simulink library "QRS_Detector_Library"  (R2021a)
settings: Solver=VariableStepAuto  StartTime=0.0  StopTime=10.0  RelTol=1e-3
undefined symbols (not defined in the file): centerFrequency, qualityFactor, sampleTime
libraries: simulink x2
settings Model: Creator=wallyproenza  LastModifiedBy=wallyproenza

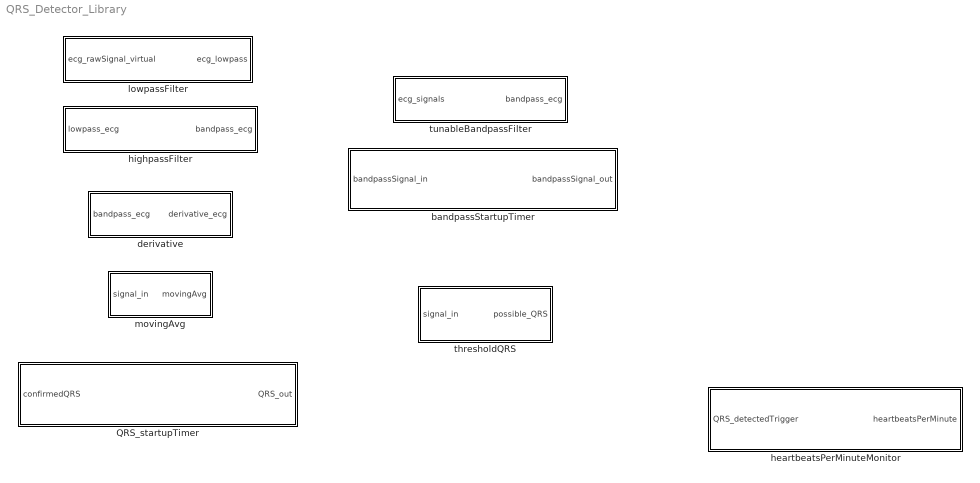
== system QRS_Detector_Library ==
  QRS_startupTimer : Subsystem
  bandpassStartupTimer : Subsystem
  derivative : Subsystem
  heartbeatsPerMinuteMonitor : Subsystem
  highpassFilter : Subsystem
  lowpassFilter : Subsystem
  movingAvg : Subsystem
  thresholdQRS : Subsystem
  tunableBandpassFilter : Subsystem

== system QRS_Detector_Library/QRS_startupTimer ==
  note: QRS startup timer helps avoid startup-related false positives
  confirmedQRS : Inport
  Cast To Double1 : DataTypeConversion  OutDataTypeStr=double
  Clock1 : Clock
  Switch1 : Switch  Criteria=u2 > Threshold  Threshold=900*sampleTime
  Zero1 : Constant  Value=0  OutDataTypeStr=Inherit: Inherit via back propagation
  QRS_out : Outport
  wires:
  confirmedQRS/1 -> Switch1/1
  Zero1/1 -> Switch1/3
  Cast To Double1/1 -> Switch1/2
  Switch1/1 -> QRS_out/1
  Clock1/1 -> Cast To Double1/1

== system QRS_Detector_Library/bandpassStartupTimer ==
  note: This bandpass startup timer helps avoids startup-related noise skew
  bandpassSignal_in : Inport
  Cast To Double : DataTypeConversion  OutDataTypeStr=double
  Clock : Clock
  Switch : Switch  Criteria=u2 > Threshold  Threshold=125*sampleTime
  Zero : Constant  Value=0  OutDataTypeStr=Inherit: Inherit via back propagation
  bandpassSignal_out : Outport
  wires:
  Cast To Double/1 -> Switch/2
  Switch/1 -> bandpassSignal_out/1
  bandpassSignal_in/1 -> Switch/1
  Zero/1 -> Switch/3
  Clock/1 -> Cast To Double/1

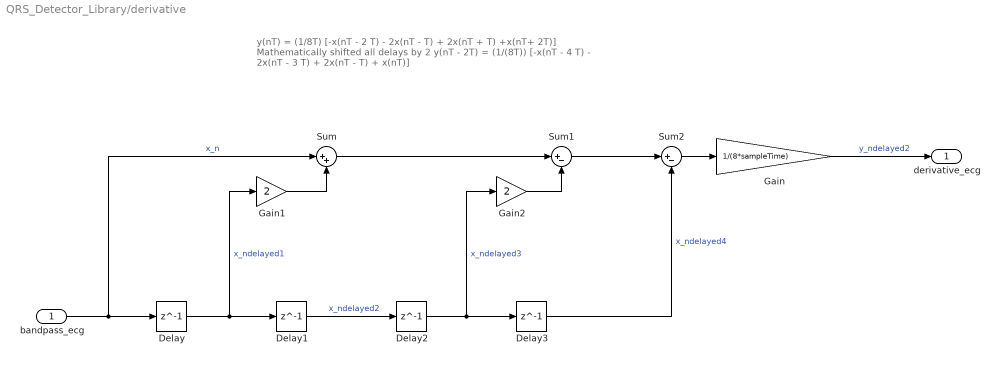
== system QRS_Detector_Library/derivative ==
  note: y(nT) = (1/8T) [-x(nT - 2 T) - 2x(nT - T) + 2x(nT + T) +x(nT+ 2T)]
      |
      | Mathematically shifted all delays by 2
      |
      | y(nT - 2T) = (1/(8T)) [-x(nT - 4 T) - 2x(nT - 3 T) + 2x(nT - T) + x(nT)]
  bandpass_ecg : Inport
  Delay{,1..3} (4 alike) : Delay  DelayLength=1  InitialCondition=0
  Gain : Gain  Gain=1/(8*sampleTime)
  Gain1 : Gain  Gain=2
  Gain2 : Gain  Gain=2
  Sum : Sum  Inputs=|++
  Sum1 : Sum  Inputs=|+-
  Sum2 : Sum  Inputs=|+-
  derivative_ecg : Outport
  wires:
  Gain/1 -> derivative_ecg/1  "y_ndelayed2"
  bandpass_ecg/1 -> Sum/1, Delay/1  "x_n"
  Delay/1 -> Gain1/1, Delay1/1  "x_ndelayed1"
  Delay1/1 -> Delay2/1  "x_ndelayed2"
  Delay2/1 -> Gain2/1, Delay3/1  "x_ndelayed3"
  Delay3/1 -> Sum2/2  "x_ndelayed4"
  Gain1/1 -> Sum/2
  Gain2/1 -> Sum1/2
  Sum/1 -> Sum1/1
  Sum1/1 -> Sum2/1
  Sum2/1 -> Gain/1

== system QRS_Detector_Library/heartbeatsPerMinuteMonitor ==
  QRS_detectedTrigger : Inport
  Cast To Double : DataTypeConversion  OutDataTypeStr=double
  Clock1 : Clock
  Compare To Constant : simulink/Logic and Bit Operations/Compare To Constant  relop=>=  const=900*sampleTime  OutDataTypeStr=boolean
  Enabled and Triggered Subsystem : Subsystem  TreatAsAtomicUnit=on
  heartbeatsPerMinute : Outport
  wires:
  QRS_detectedTrigger/1 -> Enabled and Triggered Subsystem/Trigger, Enabled and Triggered Subsystem/2(QRS_detectedTrigger)
  Clock1/1 -> Cast To Double/1
  Enabled and Triggered Subsystem/1(heartbeatsPerMinute) -> heartbeatsPerMinute/1
  Compare To Constant/1 -> Enabled and Triggered Subsystem/Enable
  Cast To Double/1 -> Enabled and Triggered Subsystem/1(clock), Compare To Constant/1

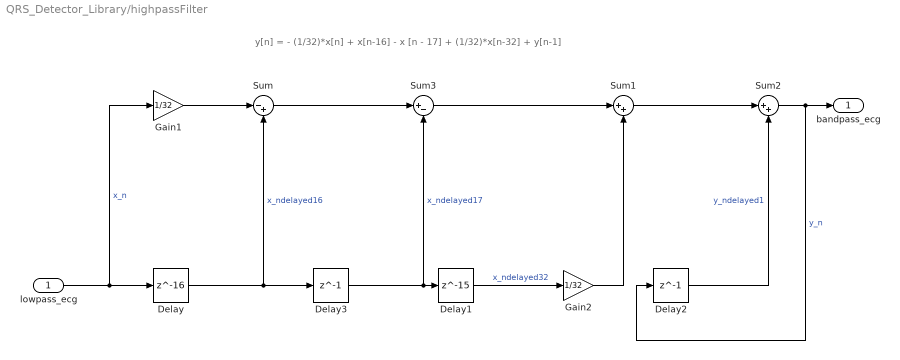
== system QRS_Detector_Library/highpassFilter ==
  note: y[n] = - (1/32)*x[n] + x[n-16] - x [n - 17] + (1/32)*x[n-32] + y[n-1]
  lowpass_ecg : Inport
  Delay : Delay  DelayLength=16  InitialCondition=0
  Delay1 : Delay  DelayLength=15  InitialCondition=0
  Delay2 : Delay  DelayLength=1  InitialCondition=0
  Delay3 : Delay  DelayLength=1  InitialCondition=0
  Gain1 : Gain  Gain=1/32
  Gain2 : Gain  Gain=1/32
  Sum : Sum  Inputs=|-+
  Sum1 : Sum  Inputs=|++
  Sum2 : Sum  Inputs=|++
  Sum3 : Sum  Inputs=|+-
  bandpass_ecg : Outport
  wires:
  lowpass_ecg/1 -> Gain1/1, Delay/1  "x_n"
  Delay/1 -> Delay3/1, Sum/2  "x_ndelayed16"
  Delay1/1 -> Gain2/1  "x_ndelayed32"
  Sum1/1 -> Sum2/1
  Delay2/1 -> Sum2/2  "y_ndelayed1"
  Sum2/1 -> Delay2/1, bandpass_ecg/1  "y_n"
  Gain1/1 -> Sum/1
  Delay3/1 -> Delay1/1, Sum3/2  "x_ndelayed17"
  Sum/1 -> Sum3/1
  Sum3/1 -> Sum1/1
  Gain2/1 -> Sum1/2

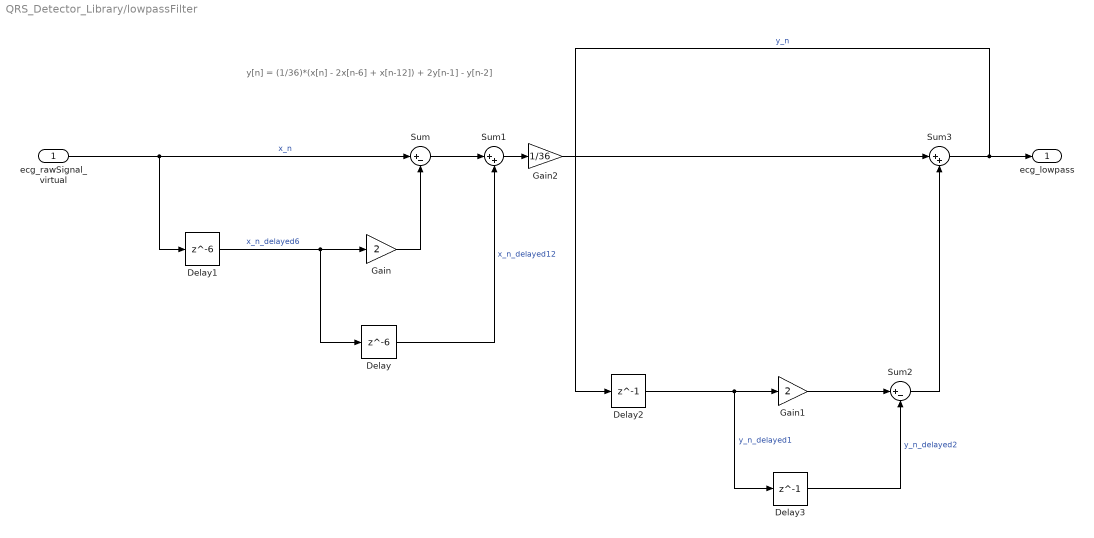
== system QRS_Detector_Library/lowpassFilter ==
  note: y[n] = (1/36)*(x[n] - 2x[n-6] + x[n-12]) + 2y[n-1] - y[n-2]
  ecg_rawSignal_virtual : Inport
  Delay : Delay  DelayLength=6  InitialCondition=0
  Delay1 : Delay  DelayLength=6  InitialCondition=0
  Delay2 : Delay  DelayLength=1  InitialCondition=0
  Delay3 : Delay  DelayLength=1  InitialCondition=0
  Gain : Gain  Gain=2
  Gain1 : Gain  Gain=2
  Gain2 : Gain  Gain=1/36
  Sum : Sum  Inputs=|+-
  Sum1 : Sum  Inputs=|++
  Sum2 : Sum  Inputs=|+-
  Sum3 : Sum  Inputs=|++
  ecg_lowpass : Outport
  wires:
  ecg_rawSignal_virtual/1 -> Delay1/1, Sum/1  "x_n"
  Delay1/1 -> Gain/1, Delay/1  "x_n_delayed6"
  Gain/1 -> Sum/2
  Delay/1 -> Sum1/2  "x_n_delayed12"
  Sum/1 -> Sum1/1
  Sum1/1 -> Gain2/1
  Delay2/1 -> Delay3/1, Gain1/1  "y_n_delayed1"
  Gain1/1 -> Sum2/1
  Delay3/1 -> Sum2/2  "y_n_delayed2"
  Sum2/1 -> Sum3/2
  Sum3/1 -> ecg_lowpass/1, Delay2/1  "y_n"
  Gain2/1 -> Sum3/1

== system QRS_Detector_Library/movingAvg ==
  signal_in : Inport
  Add : Sum  Inputs=+-+
  Constant : Constant  Value=38
  Delay : Delay  DelayLength=38  InitialCondition=0
  Delay1 : Delay  DelayLength=1  InitialCondition=0
  Divide : Product  Inputs=*/
  movingAvg : Outport
  wires:
  Constant/1 -> Divide/2
  Divide/1 -> movingAvg/1
  signal_in/1 -> Delay/1, Add/1  "x_n"
  Delay/1 -> Add/2  "x_ndelayed38"
  Add/1 -> Divide/1, Delay1/1  "currSum"
  Delay1/1 -> Add/3  "prevSum"

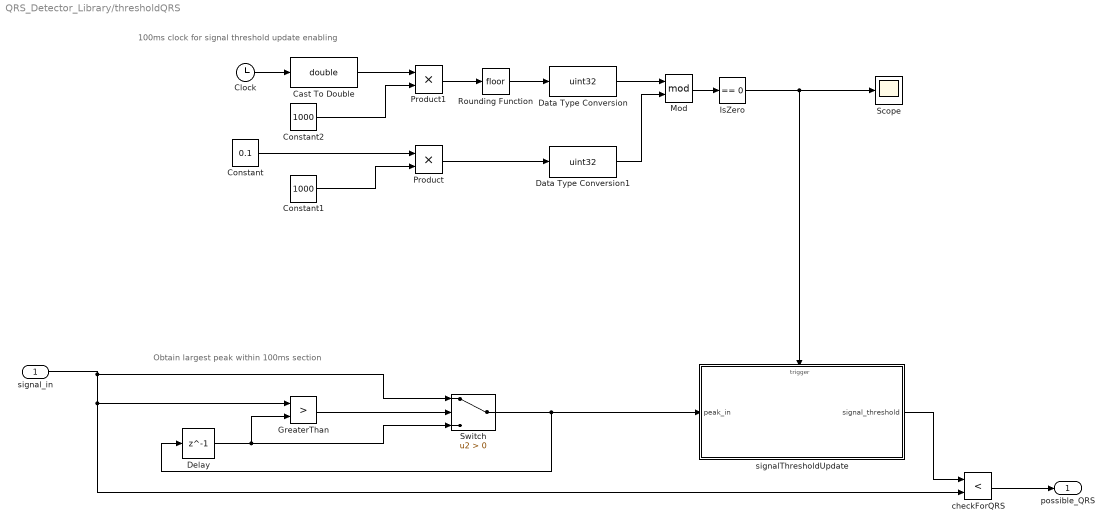
== system QRS_Detector_Library/thresholdQRS ==
  note: Obtain largest peak within 100ms section
  note: 100ms clock for signal threshold update enabling
  signal_in : Inport
  Cast To Double : DataTypeConversion  OutDataTypeStr=double
  Clock : Clock
  Constant : Constant  Value=0.1
  Constant1 : Constant  Value=1000
  Constant2 : Constant  Value=1000
  Data Type Conversion : DataTypeConversion  OutDataTypeStr=uint32
  Data Type Conversion1 : DataTypeConversion  OutDataTypeStr=uint32
  Delay : Delay  DelayLength=1  InitialCondition=0
  GreaterThan : RelationalOperator  Operator=>  OutDataTypeStr=boolean  RndMeth=Simplest
  IsZero : simulink/Logic and Bit Operations/Compare To Zero  relop===  OutDataTypeStr=boolean
  Mod : Math  Operator=mod  SaturateOnIntegerOverflow=on
  Product : Product
  Product1 : Product
  Rounding Function : Rounding
  Scope : Scope
  Switch : Switch  Criteria=u2 > Threshold
  checkForQRS : RelationalOperator  Operator=<  OutDataTypeStr=boolean  RndMeth=Simplest
  signalThresholdUpdate : Subsystem
  possible_QRS : Outport
  wires:
  signal_in/1 -> checkForQRS/2, GreaterThan/1, Switch/1
  signalThresholdUpdate/1(signal_threshold) -> checkForQRS/1
  Rounding Function/1 -> Data Type Conversion/1
  Constant/1 -> Product/1
  Product/1 -> Data Type Conversion1/1
  Constant1/1 -> Product/2
  Constant2/1 -> Product1/2
  Clock/1 -> Cast To Double/1
  Product1/1 -> Rounding Function/1
  Data Type Conversion1/1 -> Mod/2
  Data Type Conversion/1 -> Mod/1
  Mod/1 -> IsZero/1
  IsZero/1 -> signalThresholdUpdate/Trigger, Scope/1
  Cast To Double/1 -> Product1/1
  checkForQRS/1 -> possible_QRS/1
  GreaterThan/1 -> Switch/2
  Switch/1 -> Delay/1, signalThresholdUpdate/1(peak_in)
  Delay/1 -> Switch/3, GreaterThan/2

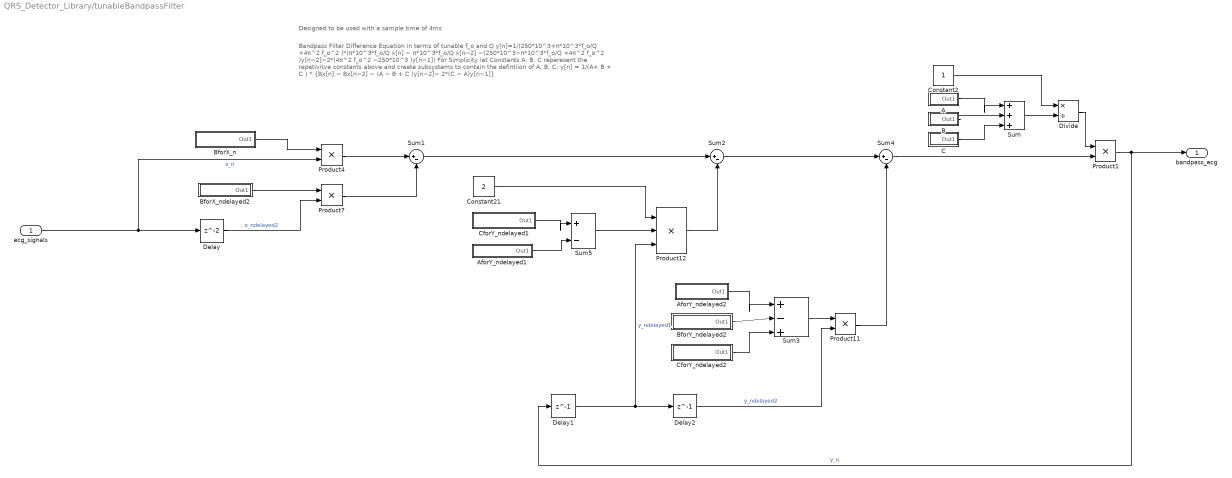
== system QRS_Detector_Library/tunableBandpassFilter ==
  note: Bandpass Filter Difference Equation in terms of tunable f_o and Q
      |
      | y[n]=1/(250*10^3+π*10^3*f_o/Q  +4π^2 f_o^2 )*(π*10^3*f_o/Q x[n]  − π*10^3*f_o/Q x[n−2]  −(250*10^3−π*10^3*f_o/Q  +4π^2 f_o^2 )y[n−2]−2*(4π^2 f_o^2  −250*10^3 )y[n−1])
      |
      |
      | For Simplicity let Constants A, B, C reperesent the repetivitve constants above and create subsystems to contain the defintiion of A, B, C:
      |
      | y[n] = 1/(A+ B + C ) * {Bx[n]  − Bx[n−2]  − (A − B + C )y[n−2]− 2*(C  − A)y[n−1]}
  note: Designed to be used with a sample time of 4ms
  ecg_signals : Inport
  A : Subsystem
  AforY_ndelayed1 : Subsystem
  AforY_ndelayed2 : Subsystem
  B : Subsystem
  BforX_n : Subsystem
  BforX_ndelayed2 : Subsystem
  BforY_ndelayed2 : Subsystem
  C : Subsystem
  CforY_ndelayed1 : Subsystem
  CforY_ndelayed2 : Subsystem
  Constant2 : Constant
  Constant21 : Constant  Value=2
  Delay : Delay  InitialCondition=0
  Delay1 : Delay  DelayLength=1  InitialCondition=0
  Delay2 : Delay  DelayLength=1  InitialCondition=0
  Divide : Product  Inputs=*/
  Product{1,4,7,11} (4 alike) : Product
  Product12 : Product  Inputs=3
  Sum : Sum  Inputs=|+++
  Sum{1..2,4..5} (4 alike) : Sum  Inputs=|+-
  Sum3 : Sum  Inputs=|+-+
  bandpass_ecg : Outport
  wires:
  ecg_signals/1 -> Product4/2, Delay/1  "x_n"
  Delay1/1 -> Product12/3, Delay2/1  "y_ndelayed1"
  Product1/1 -> Delay1/1, bandpass_ecg/1  "y_n"
  Constant2/1 -> Divide/1
  Sum/1 -> Divide/2
  Divide/1 -> Product1/1
  Product4/1 -> Sum1/1
  Product7/1 -> Sum1/2
  Delay/1 -> Product7/2  "x_ndelayed2"
  Sum1/1 -> Sum2/1
  Sum3/1 -> Product11/1
  Product11/1 -> Sum4/2
  Delay2/1 -> Product11/2  "y_ndelayed2"
  Sum4/1 -> Product1/2
  Sum2/1 -> Sum4/1
  Product12/1 -> Sum2/2
  Constant21/1 -> Product12/1
  Sum5/1 -> Product12/2
  A/1(Out1) -> Sum/1
  B/1(Out1) -> Sum/2
  C/1(Out1) -> Sum/3
  BforX_n/1(Out1) -> Product4/1
  BforX_ndelayed2/1(Out1) -> Product7/1
  AforY_ndelayed1/1(Out1) -> Sum5/2
  CforY_ndelayed1/1(Out1) -> Sum5/1
  AforY_ndelayed2/1(Out1) -> Sum3/1
  BforY_ndelayed2/1(Out1) -> Sum3/2
  CforY_ndelayed2/1(Out1) -> Sum3/3

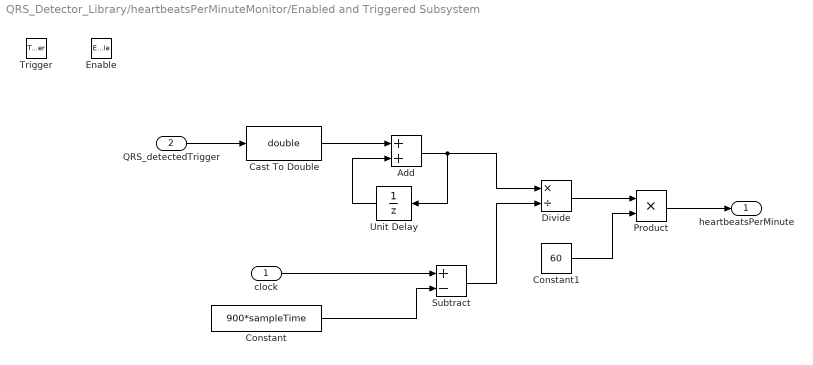
== system QRS_Detector_Library/heartbeatsPerMinuteMonitor/Enabled and Triggered Subsystem ==
  clock : Inport
  QRS_detectedTrigger : Inport  Port=2
  Enable : EnablePort
  Trigger : TriggerPort  VariantControl=(inherit)
  Add : Sum
  Cast To Double : DataTypeConversion  OutDataTypeStr=double
  Constant : Constant  Value=900*sampleTime
  Constant1 : Constant  Value=60
  Divide : Product  Inputs=*/
  Product : Product
  Subtract : Sum  Inputs=+-
  Unit Delay : UnitDelay  SampleTime=-1  HasFrameUpgradeWarning=on
  heartbeatsPerMinute : Outport
  wires:
  clock/1 -> Subtract/1
  Constant/1 -> Subtract/2
  Constant1/1 -> Product/2
  Subtract/1 -> Divide/2
  Product/1 -> heartbeatsPerMinute/1
  QRS_detectedTrigger/1 -> Cast To Double/1
  Add/1 -> Unit Delay/1, Divide/1
  Unit Delay/1 -> Add/2
  Divide/1 -> Product/1
  Cast To Double/1 -> Add/1

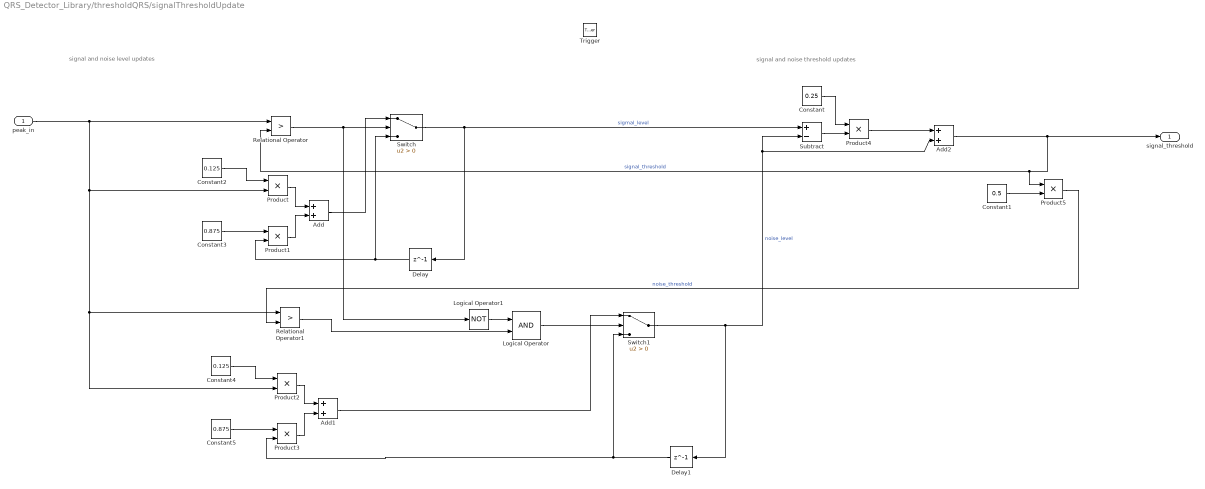
== system QRS_Detector_Library/thresholdQRS/signalThresholdUpdate ==
  note: signal and noise threshold updates
  note: signal and noise level updates
  peak_in : Inport
  Trigger : TriggerPort  VariantControl=(inherit)  PortDimensions=1
  Add : Sum
  Add1 : Sum
  Add2 : Sum
  Constant : Constant  Value=0.25
  Constant1 : Constant  Value=0.5
  Constant2 : Constant  Value=0.125
  Constant3 : Constant  Value=0.875
  Constant4 : Constant  Value=0.125
  Constant5 : Constant  Value=0.875
  Delay : Delay  DelayLength=1  InitialCondition=0
  Delay1 : Delay  DelayLength=1  InitialCondition=0
  Logical Operator : Logic  IconShape=distinctive  AllPortsSameDT=off  OutDataTypeStr=boolean
  Logical Operator1 : Logic  Operator=NOT  IconShape=distinctive  AllPortsSameDT=off  OutDataTypeStr=boolean
  Product{,1..5} (6 alike) : Product
  Relational Operator : RelationalOperator  Operator=>  OutDataTypeStr=boolean  RndMeth=Simplest
  Relational Operator1 : RelationalOperator  Operator=>  OutDataTypeStr=boolean  RndMeth=Simplest
  Subtract : Sum  Inputs=+-
  Switch : Switch  Criteria=u2 > Threshold
  Switch1 : Switch  Criteria=u2 > Threshold
  signal_threshold : Outport
  wires:
  Constant5/1 -> Product3/1
  Product3/1 -> Add1/2
  Add/1 -> Switch/1
  Product2/1 -> Add1/1
  Switch1/1 -> Delay1/1, Add2/2, Subtract/2  "noise_level"
  Product/1 -> Add/1
  Constant2/1 -> Product/1
  Constant1/1 -> Product5/2
  Add2/1 -> signal_threshold/1, Product5/1, Relational Operator/2  "signal_threshold"
  Product4/1 -> Add2/1
  Logical Operator/1 -> Switch1/2
  Constant/1 -> Product4/1
  peak_in/1 -> Relational Operator/1, Product/2, Relational Operator1/1, Product2/2
  Delay1/1 -> Product3/2, Switch1/3
  Logical Operator1/1 -> Logical Operator/1
  Constant4/1 -> Product2/1
  Delay/1 -> Switch/3, Product1/2
  Product1/1 -> Add/2
  Add1/1 -> Switch1/1
  Switch/1 -> Delay/1, Subtract/1  "sigmal_level"
  Constant3/1 -> Product1/1
  Relational Operator/1 -> Logical Operator1/1, Switch/2
  Product5/1 -> Relational Operator1/2  "noise_threshold"
  Subtract/1 -> Product4/2
  Relational Operator1/1 -> Logical Operator/2

== system QRS_Detector_Library/tunableBandpassFilter/A ==
  Constant : Constant  Value=250
  Constant1 : Constant  Value=3
  Power of 10 : Math  Operator=10^u  SaturateOnIntegerOverflow=on
  Product : Product
  Out1 : Outport
  wires:
  Power of 10/1 -> Product/2
  Constant/1 -> Product/1
  Product/1 -> Out1/1
  Constant1/1 -> Power of 10/1

== system QRS_Detector_Library/tunableBandpassFilter/AforY_ndelayed1 ==
  Constant24 : Constant  Value=250
  Constant25 : Constant  Value=3
  Power of 6 : Math  Operator=10^u  SaturateOnIntegerOverflow=on
  Product14 : Product
  Out1 : Outport
  wires:
  Product14/1 -> Out1/1
  Power of 6/1 -> Product14/2
  Constant24/1 -> Product14/1
  Constant25/1 -> Power of 6/1

== system QRS_Detector_Library/tunableBandpassFilter/AforY_ndelayed2 ==
  Constant14 : Constant  Value=250
  Constant15 : Constant  Value=3
  Power of 5 : Math  Operator=10^u  SaturateOnIntegerOverflow=on
  Product8 : Product
  Out1 : Outport
  wires:
  Constant14/1 -> Product8/1
  Product8/1 -> Out1/1
  Power of 5/1 -> Product8/2
  Constant15/1 -> Power of 5/1

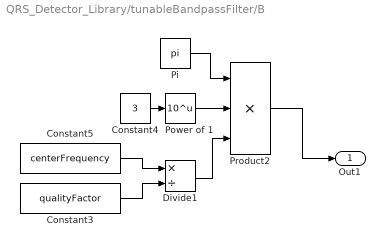
== system QRS_Detector_Library/tunableBandpassFilter/B ==
  Constant3 : Constant  Value=qualityFactor
  Constant4 : Constant  Value=3
  Constant5 : Constant  Value=centerFrequency
  Divide1 : Product  Inputs=*/
  Pi : Constant  Value=pi  OutDataTypeStr=Inherit: Inherit via back propagation
  Power of 1 : Math  Operator=10^u  SaturateOnIntegerOverflow=on
  Product2 : Product  Inputs=3
  Out1 : Outport
  wires:
  Product2/1 -> Out1/1
  Constant5/1 -> Divide1/1
  Divide1/1 -> Product2/3
  Power of 1/1 -> Product2/2
  Constant3/1 -> Divide1/2
  Pi/1 -> Product2/1
  Constant4/1 -> Power of 1/1

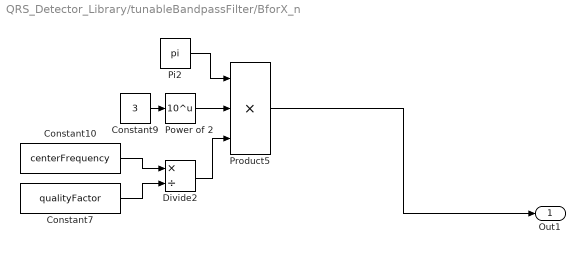
== system QRS_Detector_Library/tunableBandpassFilter/BforX_n ==
  Constant10 : Constant  Value=centerFrequency
  Constant7 : Constant  Value=qualityFactor
  Constant9 : Constant  Value=3
  Divide2 : Product  Inputs=*/
  Pi2 : Constant  Value=pi  OutDataTypeStr=Inherit: Inherit via back propagation
  Power of 2 : Math  Operator=10^u  SaturateOnIntegerOverflow=on
  Product5 : Product  Inputs=3
  Out1 : Outport
  wires:
  Product5/1 -> Out1/1
  Divide2/1 -> Product5/3
  Constant7/1 -> Divide2/2
  Constant10/1 -> Divide2/1
  Pi2/1 -> Product5/1
  Constant9/1 -> Power of 2/1
  Power of 2/1 -> Product5/2

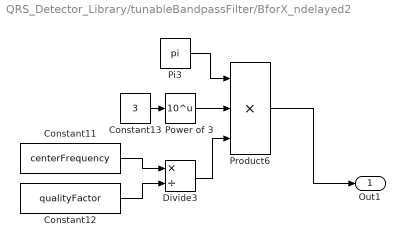
== system QRS_Detector_Library/tunableBandpassFilter/BforX_ndelayed2 ==
  Constant11 : Constant  Value=centerFrequency
  Constant12 : Constant  Value=qualityFactor
  Constant13 : Constant  Value=3
  Divide3 : Product  Inputs=*/
  Pi3 : Constant  Value=pi  OutDataTypeStr=Inherit: Inherit via back propagation
  Power of 3 : Math  Operator=10^u  SaturateOnIntegerOverflow=on
  Product6 : Product  Inputs=3
  Out1 : Outport
  wires:
  Product6/1 -> Out1/1
  Pi3/1 -> Product6/1
  Constant11/1 -> Divide3/1
  Constant12/1 -> Divide3/2
  Power of 3/1 -> Product6/2
  Constant13/1 -> Power of 3/1
  Divide3/1 -> Product6/3

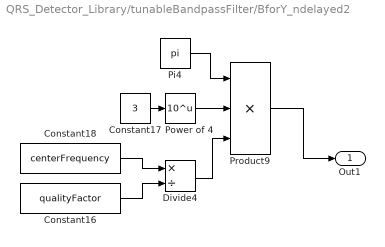
== system QRS_Detector_Library/tunableBandpassFilter/BforY_ndelayed2 ==
  Constant16 : Constant  Value=qualityFactor
  Constant17 : Constant  Value=3
  Constant18 : Constant  Value=centerFrequency
  Divide4 : Product  Inputs=*/
  Pi4 : Constant  Value=pi  OutDataTypeStr=Inherit: Inherit via back propagation
  Power of 4 : Math  Operator=10^u  SaturateOnIntegerOverflow=on
  Product9 : Product  Inputs=3
  Out1 : Outport
  wires:
  Constant18/1 -> Divide4/1
  Product9/1 -> Out1/1
  Power of 4/1 -> Product9/2
  Constant16/1 -> Divide4/2
  Divide4/1 -> Product9/3
  Pi4/1 -> Product9/1
  Constant17/1 -> Power of 4/1

== system QRS_Detector_Library/tunableBandpassFilter/C ==
  Constant6 : Constant  Value=4
  Constant8 : Constant  Value=centerFrequency
  Pi1 : Constant  Value=pi  OutDataTypeStr=Inherit: Inherit via back propagation
  Product3 : Product  Inputs=3
  Square : Math  Operator=square  SaturateOnIntegerOverflow=on
  Square1 : Math  Operator=square  SaturateOnIntegerOverflow=on
  Out1 : Outport
  wires:
  Product3/1 -> Out1/1
  Square1/1 -> Product3/3
  Square/1 -> Product3/2
  Pi1/1 -> Square/1
  Constant8/1 -> Square1/1
  Constant6/1 -> Product3/1

== system QRS_Detector_Library/tunableBandpassFilter/CforY_ndelayed1 ==
  Constant22 : Constant  Value=4
  Constant23 : Constant  Value=centerFrequency
  Pi6 : Constant  Value=pi  OutDataTypeStr=Inherit: Inherit via back propagation
  Product13 : Product  Inputs=3
  Square4 : Math  Operator=square  SaturateOnIntegerOverflow=on
  Square5 : Math  Operator=square  SaturateOnIntegerOverflow=on
  Out1 : Outport
  wires:
  Product13/1 -> Out1/1
  Square5/1 -> Product13/3
  Square4/1 -> Product13/2
  Pi6/1 -> Square4/1
  Constant22/1 -> Product13/1
  Constant23/1 -> Square5/1

== system QRS_Detector_Library/tunableBandpassFilter/CforY_ndelayed2 ==
  Constant19 : Constant  Value=4
  Constant20 : Constant  Value=centerFrequency
  Pi5 : Constant  Value=pi  OutDataTypeStr=Inherit: Inherit via back propagation
  Product10 : Product  Inputs=3
  Square2 : Math  Operator=square  SaturateOnIntegerOverflow=on
  Square3 : Math  Operator=square  SaturateOnIntegerOverflow=on
  Out1 : Outport
  wires:
  Square2/1 -> Product10/2
  Square3/1 -> Product10/3
  Product10/1 -> Out1/1
  Constant20/1 -> Square3/1
  Pi5/1 -> Square2/1
  Constant19/1 -> Product10/1
